simulink model "VCU_CS75_12_30_test"  (R2014a)
settings: Solver=FixedStepDiscrete  StartTime=0.0  StopTime=25  FixedStep=0.0005  RelTol=1e-3
InitFcn:
  | PID_canshu
values from neighbouring files (symbols this model uses):
  D1 = ecucoder_cal(D1)    [PID_canshu.m]
  D2 = ecucoder_cal(D2)    [PID_canshu.m]
  D3 = ecucoder_cal(D3)    [PID_canshu.m]
  ErrorLimit = ecucoder_cal(ErrorLimit)    [PID_canshu.m]
  ErrorSumMax1 = ecucoder_cal(ErrorSumMax1)    [PID_canshu.m]
  ErrorSumMax2 = ecucoder_cal(ErrorSumMax2)    [PID_canshu.m]
  ErrorSumMax3 = ecucoder_cal(ErrorSumMax3)    [PID_canshu.m]
  I1 = ecucoder_cal(I1)    [PID_canshu.m]
  I2 = ecucoder_cal(I2)    [PID_canshu.m]
  I3 = ecucoder_cal(I3)    [PID_canshu.m]
  Limit1 = ecucoder_cal(Limit1)    [PID_canshu.m]
  Limit2 = ecucoder_cal(Limit2)    [PID_canshu.m]
  P1 = ecucoder_cal(P1)    [PID_canshu.m]
  P2 = ecucoder_cal(P2)    [PID_canshu.m]
  P3 = ecucoder_cal(P3)    [PID_canshu.m]
  T_buchang = ecucoder_cal(T_buchang)    [PID_canshu.m]
undefined symbols (not defined in the file or in its folder): ecucoder_acal, I_SW01_L, LaterlAngleCommand, LDW, RemoteAcclPosition
libraries: simulink x940, ec5744lib x41
(part 9 of 31)

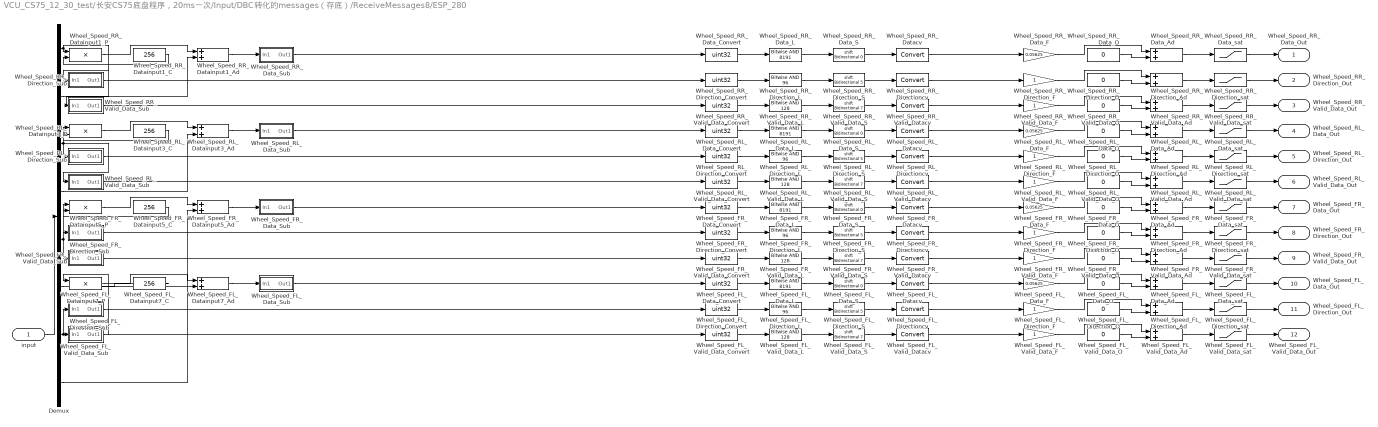
== system VCU_CS75_12_30_test/长安CS75底盘程序，20ms一次/Input/DBC转化的messages（存底）/ReceiveMessages8/ESP_280 ==
  input : Inport
  Demux : Demux  Outputs=8
  Wheel_Speed_FL_Data_Ad : Sum
  Wheel_Speed_FL_Data_Convert : DataTypeConversion  OutDataTypeStr=uint32
  Wheel_Speed_FL_Data_F : Gain  Gain=0.05625
  Wheel_Speed_FL_Data_L : simulink/Logic and Bit Operations/Bitwise Operator  logicop=AND  UseBitMask=on  BitMask=8191  BitMaskRealWorld=Stored Integer
  Wheel_Speed_FL_Data_O : Constant  Value=0  OutDataTypeStr=single
  Wheel_Speed_FL_Data_S : ArithShift
  Wheel_Speed_FL_Data_Sub : Subsystem
  Wheel_Speed_FL_Data_sat : Saturate  UpperLimit=360  LowerLimit=0
  Wheel_Speed_FL_Datacv : DataTypeConversion
  Wheel_Speed_FL_Datainput7_Ad : Sum
  Wheel_Speed_FL_Datainput7_C : Constant  Value=256
  Wheel_Speed_FL_Datainput7_P : Product
  Wheel_Speed_FL_Direction_Ad : Sum
  Wheel_Speed_FL_Direction_Convert : DataTypeConversion  OutDataTypeStr=uint32
  Wheel_Speed_FL_Direction_F : Gain
  Wheel_Speed_FL_Direction_L : simulink/Logic and Bit Operations/Bitwise Operator  logicop=AND  UseBitMask=on  BitMask=96  BitMaskRealWorld=Stored Integer
  Wheel_Speed_FL_Direction_O : Constant  Value=0  OutDataTypeStr=single
  Wheel_Speed_FL_Direction_S : ArithShift  BitShiftNumber=5
  Wheel_Speed_FL_Direction_Sub : Subsystem
  Wheel_Speed_FL_Direction_sat : Saturate  UpperLimit=3  LowerLimit=0
  Wheel_Speed_FL_Directioncv : DataTypeConversion
  Wheel_Speed_FL_Valid_Data_Ad : Sum
  Wheel_Speed_FL_Valid_Data_Convert : DataTypeConversion  OutDataTypeStr=uint32
  Wheel_Speed_FL_Valid_Data_F : Gain
  Wheel_Speed_FL_Valid_Data_L : simulink/Logic and Bit Operations/Bitwise Operator  logicop=AND  UseBitMask=on  BitMask=128  BitMaskRealWorld=Stored Integer
  Wheel_Speed_FL_Valid_Data_O : Constant  Value=0  OutDataTypeStr=single
  Wheel_Speed_FL_Valid_Data_S : ArithShift  BitShiftNumber=7
  Wheel_Speed_FL_Valid_Data_Sub : Subsystem
  Wheel_Speed_FL_Valid_Data_sat : Saturate  UpperLimit=1  LowerLimit=0
  Wheel_Speed_FL_Valid_Datacv : DataTypeConversion
  Wheel_Speed_FR_Data_Ad : Sum
  Wheel_Speed_FR_Data_Convert : DataTypeConversion  OutDataTypeStr=uint32
  Wheel_Speed_FR_Data_F : Gain  Gain=0.05625
  Wheel_Speed_FR_Data_L : simulink/Logic and Bit Operations/Bitwise Operator  logicop=AND  UseBitMask=on  BitMask=8191  BitMaskRealWorld=Stored Integer
  Wheel_Speed_FR_Data_O : Constant  Value=0  OutDataTypeStr=single
  Wheel_Speed_FR_Data_S : ArithShift
  Wheel_Speed_FR_Data_Sub : Subsystem
  Wheel_Speed_FR_Data_sat : Saturate  UpperLimit=360  LowerLimit=0
  Wheel_Speed_FR_Datacv : DataTypeConversion
  Wheel_Speed_FR_Datainput5_Ad : Sum
  Wheel_Speed_FR_Datainput5_C : Constant  Value=256
  Wheel_Speed_FR_Datainput5_P : Product
  Wheel_Speed_FR_Direction_Ad : Sum
  Wheel_Speed_FR_Direction_Convert : DataTypeConversion  OutDataTypeStr=uint32
  Wheel_Speed_FR_Direction_F : Gain
  Wheel_Speed_FR_Direction_L : simulink/Logic and Bit Operations/Bitwise Operator  logicop=AND  UseBitMask=on  BitMask=96  BitMaskRealWorld=Stored Integer
  Wheel_Speed_FR_Direction_O : Constant  Value=0  OutDataTypeStr=single
  Wheel_Speed_FR_Direction_S : ArithShift  BitShiftNumber=5
  Wheel_Speed_FR_Direction_Sub : Subsystem
  Wheel_Speed_FR_Direction_sat : Saturate  UpperLimit=3  LowerLimit=0
  Wheel_Speed_FR_Directioncv : DataTypeConversion
  Wheel_Speed_FR_Valid_Data_Ad : Sum
  Wheel_Speed_FR_Valid_Data_Convert : DataTypeConversion  OutDataTypeStr=uint32
  Wheel_Speed_FR_Valid_Data_F : Gain
  Wheel_Speed_FR_Valid_Data_L : simulink/Logic and Bit Operations/Bitwise Operator  logicop=AND  UseBitMask=on  BitMask=128  BitMaskRealWorld=Stored Integer
  Wheel_Speed_FR_Valid_Data_O : Constant  Value=0  OutDataTypeStr=single
  Wheel_Speed_FR_Valid_Data_S : ArithShift  BitShiftNumber=7
  Wheel_Speed_FR_Valid_Data_Sub : Subsystem
  Wheel_Speed_FR_Valid_Data_sat : Saturate  UpperLimit=1  LowerLimit=0
  Wheel_Speed_FR_Valid_Datacv : DataTypeConversion
  Wheel_Speed_RL_Data_Ad : Sum
  Wheel_Speed_RL_Data_Convert : DataTypeConversion  OutDataTypeStr=uint32
  Wheel_Speed_RL_Data_F : Gain  Gain=0.05625
  Wheel_Speed_RL_Data_L : simulink/Logic and Bit Operations/Bitwise Operator  logicop=AND  UseBitMask=on  BitMask=8191  BitMaskRealWorld=Stored Integer
  Wheel_Speed_RL_Data_O : Constant  Value=0  OutDataTypeStr=single
  Wheel_Speed_RL_Data_S : ArithShift
  Wheel_Speed_RL_Data_Sub : Subsystem
  Wheel_Speed_RL_Data_sat : Saturate  UpperLimit=360  LowerLimit=0
  Wheel_Speed_RL_Datacv : DataTypeConversion
  Wheel_Speed_RL_Datainput3_Ad : Sum
  Wheel_Speed_RL_Datainput3_C : Constant  Value=256
  Wheel_Speed_RL_Datainput3_P : Product
  Wheel_Speed_RL_Direction_Ad : Sum
  Wheel_Speed_RL_Direction_Convert : DataTypeConversion  OutDataTypeStr=uint32
  Wheel_Speed_RL_Direction_F : Gain
  Wheel_Speed_RL_Direction_L : simulink/Logic and Bit Operations/Bitwise Operator  logicop=AND  UseBitMask=on  BitMask=96  BitMaskRealWorld=Stored Integer
  Wheel_Speed_RL_Direction_O : Constant  Value=0  OutDataTypeStr=single
  Wheel_Speed_RL_Direction_S : ArithShift  BitShiftNumber=5
  Wheel_Speed_RL_Direction_Sub : Subsystem
  Wheel_Speed_RL_Direction_sat : Saturate  UpperLimit=3  LowerLimit=0
  Wheel_Speed_RL_Directioncv : DataTypeConversion
  Wheel_Speed_RL_Valid_Data_Ad : Sum
  Wheel_Speed_RL_Valid_Data_Convert : DataTypeConversion  OutDataTypeStr=uint32
  Wheel_Speed_RL_Valid_Data_F : Gain
  Wheel_Speed_RL_Valid_Data_L : simulink/Logic and Bit Operations/Bitwise Operator  logicop=AND  UseBitMask=on  BitMask=128  BitMaskRealWorld=Stored Integer
  Wheel_Speed_RL_Valid_Data_O : Constant  Value=0  OutDataTypeStr=single
  Wheel_Speed_RL_Valid_Data_S : ArithShift  BitShiftNumber=7
  Wheel_Speed_RL_Valid_Data_Sub : Subsystem
  Wheel_Speed_RL_Valid_Data_sat : Saturate  UpperLimit=1  LowerLimit=0
  Wheel_Speed_RL_Valid_Datacv : DataTypeConversion
  Wheel_Speed_RR_Data_Ad : Sum
  Wheel_Speed_RR_Data_Convert : DataTypeConversion  OutDataTypeStr=uint32
  Wheel_Speed_RR_Data_F : Gain  Gain=0.05625
  Wheel_Speed_RR_Data_L : simulink/Logic and Bit Operations/Bitwise Operator  logicop=AND  UseBitMask=on  BitMask=8191  BitMaskRealWorld=Stored Integer
  Wheel_Speed_RR_Data_O : Constant  Value=0  OutDataTypeStr=single
  Wheel_Speed_RR_Data_S : ArithShift
  Wheel_Speed_RR_Data_Sub : Subsystem
  Wheel_Speed_RR_Data_sat : Saturate  UpperLimit=360  LowerLimit=0
  Wheel_Speed_RR_Datacv : DataTypeConversion
  Wheel_Speed_RR_Datainput1_Ad : Sum
  Wheel_Speed_RR_Datainput1_C : Constant  Value=256
  Wheel_Speed_RR_Datainput1_P : Product
  Wheel_Speed_RR_Direction_Ad : Sum
  Wheel_Speed_RR_Direction_Convert : DataTypeConversion  OutDataTypeStr=uint32
  Wheel_Speed_RR_Direction_F : Gain
  Wheel_Speed_RR_Direction_L : simulink/Logic and Bit Operations/Bitwise Operator  logicop=AND  UseBitMask=on  BitMask=96  BitMaskRealWorld=Stored Integer
  Wheel_Speed_RR_Direction_O : Constant  Value=0  OutDataTypeStr=single
  Wheel_Speed_RR_Direction_S : ArithShift  BitShiftNumber=5
  Wheel_Speed_RR_Direction_Sub : Subsystem
  Wheel_Speed_RR_Direction_sat : Saturate  UpperLimit=3  LowerLimit=0
  Wheel_Speed_RR_Directioncv : DataTypeConversion
  Wheel_Speed_RR_Valid_Data_Ad : Sum
  Wheel_Speed_RR_Valid_Data_Convert : DataTypeConversion  OutDataTypeStr=uint32
  Wheel_Speed_RR_Valid_Data_F : Gain
  Wheel_Speed_RR_Valid_Data_L : simulink/Logic and Bit Operations/Bitwise Operator  logicop=AND  UseBitMask=on  BitMask=128  BitMaskRealWorld=Stored Integer
  Wheel_Speed_RR_Valid_Data_O : Constant  Value=0  OutDataTypeStr=single
  Wheel_Speed_RR_Valid_Data_S : ArithShift  BitShiftNumber=7
  Wheel_Speed_RR_Valid_Data_Sub : Subsystem
  Wheel_Speed_RR_Valid_Data_sat : Saturate  UpperLimit=1  LowerLimit=0
  Wheel_Speed_RR_Valid_Datacv : DataTypeConversion
  Wheel_Speed_RR_Data_Out : Outport
  Wheel_Speed_RR_Direction_Out : Outport  Port=2
  Wheel_Speed_RR_Valid_Data_Out : Outport  Port=3
  Wheel_Speed_RL_Data_Out : Outport  Port=4
  Wheel_Speed_RL_Direction_Out : Outport  Port=5
  Wheel_Speed_RL_Valid_Data_Out : Outport  Port=6
  Wheel_Speed_FR_Data_Out : Outport  Port=7
  Wheel_Speed_FR_Direction_Out : Outport  Port=8
  Wheel_Speed_FR_Valid_Data_Out : Outport  Port=9
  Wheel_Speed_FL_Data_Out : Outport  Port=10
  Wheel_Speed_FL_Direction_Out : Outport  Port=11
  Wheel_Speed_FL_Valid_Data_Out : Outport  Port=12
  wires:
  input/1 -> Demux/1
  Wheel_Speed_FL_Valid_Datacv/1 -> Wheel_Speed_FL_Valid_Data_F/1
  Wheel_Speed_FL_Valid_Data_S/1 -> Wheel_Speed_FL_Valid_Datacv/1
  Wheel_Speed_FL_Valid_Data_L/1 -> Wheel_Speed_FL_Valid_Data_S/1
  Wheel_Speed_FL_Valid_Data_Convert/1 -> Wheel_Speed_FL_Valid_Data_L/1
  Wheel_Speed_FL_Valid_Data_Sub/1(Out1) -> Wheel_Speed_FL_Valid_Data_Convert/1
  Wheel_Speed_FL_Valid_Data_sat/1 -> Wheel_Speed_FL_Valid_Data_Out/1
  Wheel_Speed_FL_Valid_Data_Ad/1 -> Wheel_Speed_FL_Valid_Data_sat/1
  Wheel_Speed_FL_Valid_Data_O/1 -> Wheel_Speed_FL_Valid_Data_Ad/2
  Wheel_Speed_FL_Valid_Data_F/1 -> Wheel_Speed_FL_Valid_Data_Ad/1
  Wheel_Speed_FL_Directioncv/1 -> Wheel_Speed_FL_Direction_F/1
  Wheel_Speed_FL_Direction_S/1 -> Wheel_Speed_FL_Directioncv/1
  Wheel_Speed_FL_Direction_L/1 -> Wheel_Speed_FL_Direction_S/1
  Wheel_Speed_FL_Direction_Convert/1 -> Wheel_Speed_FL_Direction_L/1
  Wheel_Speed_FL_Direction_Sub/1(Out1) -> Wheel_Speed_FL_Direction_Convert/1
  Wheel_Speed_FL_Direction_sat/1 -> Wheel_Speed_FL_Direction_Out/1
  Wheel_Speed_FL_Direction_Ad/1 -> Wheel_Speed_FL_Direction_sat/1
  Wheel_Speed_FL_Direction_O/1 -> Wheel_Speed_FL_Direction_Ad/2
  Wheel_Speed_FL_Direction_F/1 -> Wheel_Speed_FL_Direction_Ad/1
  Wheel_Speed_FL_Datacv/1 -> Wheel_Speed_FL_Data_F/1
  Wheel_Speed_FL_Data_S/1 -> Wheel_Speed_FL_Datacv/1
  Wheel_Speed_FL_Data_L/1 -> Wheel_Speed_FL_Data_S/1
  Wheel_Speed_FL_Data_Convert/1 -> Wheel_Speed_FL_Data_L/1
  Wheel_Speed_FL_Data_Sub/1(Out1) -> Wheel_Speed_FL_Data_Convert/1
  Wheel_Speed_FL_Datainput7_Ad/1 -> Wheel_Speed_FL_Data_Sub/1(In1)
  Demux/8 -> Wheel_Speed_FL_Datainput7_Ad/2
  Wheel_Speed_FL_Datainput7_P/1 -> Wheel_Speed_FL_Datainput7_Ad/1
  Wheel_Speed_FL_Datainput7_C/1 -> Wheel_Speed_FL_Datainput7_P/2
  Demux/7 -> Wheel_Speed_FL_Valid_Data_Sub/1(In1), Wheel_Speed_FL_Direction_Sub/1(In1), Wheel_Speed_FL_Datainput7_P/1
  Wheel_Speed_FL_Data_sat/1 -> Wheel_Speed_FL_Data_Out/1
  Wheel_Speed_FL_Data_Ad/1 -> Wheel_Speed_FL_Data_sat/1
  Wheel_Speed_FL_Data_O/1 -> Wheel_Speed_FL_Data_Ad/2
  Wheel_Speed_FL_Data_F/1 -> Wheel_Speed_FL_Data_Ad/1
  Wheel_Speed_FR_Valid_Datacv/1 -> Wheel_Speed_FR_Valid_Data_F/1
  Wheel_Speed_FR_Valid_Data_S/1 -> Wheel_Speed_FR_Valid_Datacv/1
  Wheel_Speed_FR_Valid_Data_L/1 -> Wheel_Speed_FR_Valid_Data_S/1
  Wheel_Speed_FR_Valid_Data_Convert/1 -> Wheel_Speed_FR_Valid_Data_L/1
  Wheel_Speed_FR_Valid_Data_Sub/1(Out1) -> Wheel_Speed_FR_Valid_Data_Convert/1
  Wheel_Speed_FR_Valid_Data_sat/1 -> Wheel_Speed_FR_Valid_Data_Out/1
  Wheel_Speed_FR_Valid_Data_Ad/1 -> Wheel_Speed_FR_Valid_Data_sat/1
  Wheel_Speed_FR_Valid_Data_O/1 -> Wheel_Speed_FR_Valid_Data_Ad/2
  Wheel_Speed_FR_Valid_Data_F/1 -> Wheel_Speed_FR_Valid_Data_Ad/1
  Wheel_Speed_FR_Directioncv/1 -> Wheel_Speed_FR_Direction_F/1
  Wheel_Speed_FR_Direction_S/1 -> Wheel_Speed_FR_Directioncv/1
  Wheel_Speed_FR_Direction_L/1 -> Wheel_Speed_FR_Direction_S/1
  Wheel_Speed_FR_Direction_Convert/1 -> Wheel_Speed_FR_Direction_L/1
  Wheel_Speed_FR_Direction_Sub/1(Out1) -> Wheel_Speed_FR_Direction_Convert/1
  Wheel_Speed_FR_Direction_sat/1 -> Wheel_Speed_FR_Direction_Out/1
  Wheel_Speed_FR_Direction_Ad/1 -> Wheel_Speed_FR_Direction_sat/1
  Wheel_Speed_FR_Direction_O/1 -> Wheel_Speed_FR_Direction_Ad/2
  Wheel_Speed_FR_Direction_F/1 -> Wheel_Speed_FR_Direction_Ad/1
  Wheel_Speed_FR_Datacv/1 -> Wheel_Speed_FR_Data_F/1
  Wheel_Speed_FR_Data_S/1 -> Wheel_Speed_FR_Datacv/1
  Wheel_Speed_FR_Data_L/1 -> Wheel_Speed_FR_Data_S/1
  Wheel_Speed_FR_Data_Convert/1 -> Wheel_Speed_FR_Data_L/1
  Wheel_Speed_FR_Data_Sub/1(Out1) -> Wheel_Speed_FR_Data_Convert/1
  Wheel_Speed_FR_Datainput5_Ad/1 -> Wheel_Speed_FR_Data_Sub/1(In1)
  Demux/6 -> Wheel_Speed_FR_Datainput5_Ad/2
  Wheel_Speed_FR_Datainput5_P/1 -> Wheel_Speed_FR_Datainput5_Ad/1
  Wheel_Speed_FR_Datainput5_C/1 -> Wheel_Speed_FR_Datainput5_P/2
  Demux/5 -> Wheel_Speed_FR_Valid_Data_Sub/1(In1), Wheel_Speed_FR_Direction_Sub/1(In1), Wheel_Speed_FR_Datainput5_P/1
  Wheel_Speed_FR_Data_sat/1 -> Wheel_Speed_FR_Data_Out/1
  Wheel_Speed_FR_Data_Ad/1 -> Wheel_Speed_FR_Data_sat/1
  Wheel_Speed_FR_Data_O/1 -> Wheel_Speed_FR_Data_Ad/2
  Wheel_Speed_FR_Data_F/1 -> Wheel_Speed_FR_Data_Ad/1
  Wheel_Speed_RL_Valid_Datacv/1 -> Wheel_Speed_RL_Valid_Data_F/1
  Wheel_Speed_RL_Valid_Data_S/1 -> Wheel_Speed_RL_Valid_Datacv/1
  Wheel_Speed_RL_Valid_Data_L/1 -> Wheel_Speed_RL_Valid_Data_S/1
  Wheel_Speed_RL_Valid_Data_Convert/1 -> Wheel_Speed_RL_Valid_Data_L/1
  Wheel_Speed_RL_Valid_Data_Sub/1(Out1) -> Wheel_Speed_RL_Valid_Data_Convert/1
  Wheel_Speed_RL_Valid_Data_sat/1 -> Wheel_Speed_RL_Valid_Data_Out/1
  Wheel_Speed_RL_Valid_Data_Ad/1 -> Wheel_Speed_RL_Valid_Data_sat/1
  Wheel_Speed_RL_Valid_Data_O/1 -> Wheel_Speed_RL_Valid_Data_Ad/2
  Wheel_Speed_RL_Valid_Data_F/1 -> Wheel_Speed_RL_Valid_Data_Ad/1
  Wheel_Speed_RL_Directioncv/1 -> Wheel_Speed_RL_Direction_F/1
  Wheel_Speed_RL_Direction_S/1 -> Wheel_Speed_RL_Directioncv/1
  Wheel_Speed_RL_Direction_L/1 -> Wheel_Speed_RL_Direction_S/1
  Wheel_Speed_RL_Direction_Convert/1 -> Wheel_Speed_RL_Direction_L/1
  Wheel_Speed_RL_Direction_Sub/1(Out1) -> Wheel_Speed_RL_Direction_Convert/1
  Wheel_Speed_RL_Direction_sat/1 -> Wheel_Speed_RL_Direction_Out/1
  Wheel_Speed_RL_Direction_Ad/1 -> Wheel_Speed_RL_Direction_sat/1
  Wheel_Speed_RL_Direction_O/1 -> Wheel_Speed_RL_Direction_Ad/2
  Wheel_Speed_RL_Direction_F/1 -> Wheel_Speed_RL_Direction_Ad/1
  Wheel_Speed_RL_Datacv/1 -> Wheel_Speed_RL_Data_F/1
  Wheel_Speed_RL_Data_S/1 -> Wheel_Speed_RL_Datacv/1
  Wheel_Speed_RL_Data_L/1 -> Wheel_Speed_RL_Data_S/1
  Wheel_Speed_RL_Data_Convert/1 -> Wheel_Speed_RL_Data_L/1
  Wheel_Speed_RL_Data_Sub/1(Out1) -> Wheel_Speed_RL_Data_Convert/1
  Wheel_Speed_RL_Datainput3_Ad/1 -> Wheel_Speed_RL_Data_Sub/1(In1)
  Demux/4 -> Wheel_Speed_RL_Datainput3_Ad/2
  Wheel_Speed_RL_Datainput3_P/1 -> Wheel_Speed_RL_Datainput3_Ad/1
  Wheel_Speed_RL_Datainput3_C/1 -> Wheel_Speed_RL_Datainput3_P/2
  Demux/3 -> Wheel_Speed_RL_Valid_Data_Sub/1(In1), Wheel_Speed_RL_Direction_Sub/1(In1), Wheel_Speed_RL_Datainput3_P/1
  Wheel_Speed_RL_Data_sat/1 -> Wheel_Speed_RL_Data_Out/1
  Wheel_Speed_RL_Data_Ad/1 -> Wheel_Speed_RL_Data_sat/1
  Wheel_Speed_RL_Data_O/1 -> Wheel_Speed_RL_Data_Ad/2
  Wheel_Speed_RL_Data_F/1 -> Wheel_Speed_RL_Data_Ad/1
  Wheel_Speed_RR_Valid_Datacv/1 -> Wheel_Speed_RR_Valid_Data_F/1
  Wheel_Speed_RR_Valid_Data_S/1 -> Wheel_Speed_RR_Valid_Datacv/1
  Wheel_Speed_RR_Valid_Data_L/1 -> Wheel_Speed_RR_Valid_Data_S/1
  Wheel_Speed_RR_Valid_Data_Convert/1 -> Wheel_Speed_RR_Valid_Data_L/1
  Wheel_Speed_RR_Valid_Data_Sub/1(Out1) -> Wheel_Speed_RR_Valid_Data_Convert/1
  Wheel_Speed_RR_Valid_Data_sat/1 -> Wheel_Speed_RR_Valid_Data_Out/1
  Wheel_Speed_RR_Valid_Data_Ad/1 -> Wheel_Speed_RR_Valid_Data_sat/1
  Wheel_Speed_RR_Valid_Data_O/1 -> Wheel_Speed_RR_Valid_Data_Ad/2
  Wheel_Speed_RR_Valid_Data_F/1 -> Wheel_Speed_RR_Valid_Data_Ad/1
  Wheel_Speed_RR_Directioncv/1 -> Wheel_Speed_RR_Direction_F/1
  Wheel_Speed_RR_Direction_S/1 -> Wheel_Speed_RR_Directioncv/1
  Wheel_Speed_RR_Direction_L/1 -> Wheel_Speed_RR_Direction_S/1
  Wheel_Speed_RR_Direction_Convert/1 -> Wheel_Speed_RR_Direction_L/1
  Wheel_Speed_RR_Direction_Sub/1(Out1) -> Wheel_Speed_RR_Direction_Convert/1
  Wheel_Speed_RR_Direction_sat/1 -> Wheel_Speed_RR_Direction_Out/1
  Wheel_Speed_RR_Direction_Ad/1 -> Wheel_Speed_RR_Direction_sat/1
  Wheel_Speed_RR_Direction_O/1 -> Wheel_Speed_RR_Direction_Ad/2
  Wheel_Speed_RR_Direction_F/1 -> Wheel_Speed_RR_Direction_Ad/1
  Wheel_Speed_RR_Datacv/1 -> Wheel_Speed_RR_Data_F/1
  Wheel_Speed_RR_Data_S/1 -> Wheel_Speed_RR_Datacv/1
  Wheel_Speed_RR_Data_L/1 -> Wheel_Speed_RR_Data_S/1
  Wheel_Speed_RR_Data_Convert/1 -> Wheel_Speed_RR_Data_L/1
  Wheel_Speed_RR_Data_Sub/1(Out1) -> Wheel_Speed_RR_Data_Convert/1
  Wheel_Speed_RR_Datainput1_Ad/1 -> Wheel_Speed_RR_Data_Sub/1(In1)
  Demux/2 -> Wheel_Speed_RR_Datainput1_Ad/2
  Wheel_Speed_RR_Datainput1_P/1 -> Wheel_Speed_RR_Datainput1_Ad/1
  Wheel_Speed_RR_Datainput1_C/1 -> Wheel_Speed_RR_Datainput1_P/2
  Demux/1 -> Wheel_Speed_RR_Valid_Data_Sub/1(In1), Wheel_Speed_RR_Direction_Sub/1(In1), Wheel_Speed_RR_Datainput1_P/1
  Wheel_Speed_RR_Data_sat/1 -> Wheel_Speed_RR_Data_Out/1
  Wheel_Speed_RR_Data_Ad/1 -> Wheel_Speed_RR_Data_sat/1
  Wheel_Speed_RR_Data_O/1 -> Wheel_Speed_RR_Data_Ad/2
  Wheel_Speed_RR_Data_F/1 -> Wheel_Speed_RR_Data_Ad/1

== system VCU_CS75_12_30_test/长安CS75底盘程序，20ms一次/Input/DBC转化的messages（存底）/ReceiveMessages9/ESP_281 ==
  input : Inport
  Demux : Demux  Outputs=8
  ESP_ABSActiveStatus_Ad : Sum
  ESP_ABSActiveStatus_Convert : DataTypeConversion  OutDataTypeStr=uint32
  ESP_ABSActiveStatus_F : Gain
  ESP_ABSActiveStatus_L : simulink/Logic and Bit Operations/Bitwise Operator  logicop=AND  UseBitMask=on  BitMask=128  BitMaskRealWorld=Stored Integer
  ESP_ABSActiveStatus_O : Constant  Value=0  OutDataTypeStr=single
  ESP_ABSActiveStatus_S : ArithShift  BitShiftNumber=7
  ESP_ABSActiveStatus_Sub : Subsystem
  ESP_ABSActiveStatus_sat : Saturate  UpperLimit=1  LowerLimit=0
  ESP_ABSActiveStatuscv : DataTypeConversion
  ESP_ABSFailStatus_Ad : Sum
  ESP_ABSFailStatus_Convert : DataTypeConversion  OutDataTypeStr=uint32
  ESP_ABSFailStatus_F : Gain
  ESP_ABSFailStatus_L : simulink/Logic and Bit Operations/Bitwise Operator  logicop=AND  UseBitMask=on  BitMask=8  BitMaskRealWorld=Stored Integer
  ESP_ABSFailStatus_O : Constant  Value=0  OutDataTypeStr=single
  ESP_ABSFailStatus_S : ArithShift  BitShiftNumber=3
  ESP_ABSFailStatus_Sub : Subsystem
  ESP_ABSFailStatus_sat : Saturate  UpperLimit=1  LowerLimit=0
  ESP_ABSFailStatuscv : DataTypeConversion
  ESP_BrakePedalStatus_Ad : Sum
  ESP_BrakePedalStatus_Convert : DataTypeConversion  OutDataTypeStr=uint32
  ESP_BrakePedalStatus_F : Gain
  ESP_BrakePedalStatus_L : simulink/Logic and Bit Operations/Bitwise Operator  logicop=AND  UseBitMask=on  BitMask=96  BitMaskRealWorld=Stored Integer
  ESP_BrakePedalStatus_O : Constant  Value=0  OutDataTypeStr=single
  ESP_BrakePedalStatus_S : ArithShift  BitShiftNumber=5
  ESP_BrakePedalStatus_Sub : Subsystem
  ESP_BrakePedalStatus_sat : Saturate  UpperLimit=3  LowerLimit=0
  ESP_BrakePedalStatuscv : DataTypeConversion
  ESP_Checksum_Ad : Sum
  ESP_Checksum_Convert : DataTypeConversion  OutDataTypeStr=uint32
  ESP_Checksum_F : Gain
  ESP_Checksum_L : simulink/Logic and Bit Operations/Bitwise Operator  logicop=AND  UseBitMask=on  BitMask=255  BitMaskRealWorld=Stored Integer
  ESP_Checksum_O : Constant  Value=0  OutDataTypeStr=single
  ESP_Checksum_S : ArithShift
  ESP_Checksum_Sub : Subsystem
  ESP_Checksum_sat : Saturate  UpperLimit=255  LowerLimit=0
  ESP_Checksumcv : DataTypeConversion
  ESP_EBDFailStatus_Ad : Sum
  ESP_EBDFailStatus_Convert : DataTypeConversion  OutDataTypeStr=uint32
  ESP_EBDFailStatus_F : Gain
  ESP_EBDFailStatus_L : simulink/Logic and Bit Operations/Bitwise Operator  logicop=AND  UseBitMask=on  BitMask=4  BitMaskRealWorld=Stored Integer
  ESP_EBDFailStatus_O : Constant  Value=0  OutDataTypeStr=single
  ESP_EBDFailStatus_S : ArithShift  BitShiftNumber=2
  ESP_EBDFailStatus_Sub : Subsystem
  ESP_EBDFailStatus_sat : Saturate  UpperLimit=1  LowerLimit=0
  ESP_EBDFailStatuscv : DataTypeConversion
  ESP_ESPActiveStatus_Ad : Sum
  ESP_ESPActiveStatus_Convert : DataTypeConversion  OutDataTypeStr=uint32
  ESP_ESPActiveStatus_F : Gain
  ESP_ESPActiveStatus_L : simulink/Logic and Bit Operations/Bitwise Operator  logicop=AND  UseBitMask=on  BitMask=1  BitMaskRealWorld=Stored Integer
  ESP_ESPActiveStatus_O : Constant  Value=0  OutDataTypeStr=single
  ESP_ESPActiveStatus_S : ArithShift
  ESP_ESPActiveStatus_Sub : Subsystem
  ESP_ESPActiveStatus_sat : Saturate  UpperLimit=1  LowerLimit=0
  ESP_ESPActiveStatuscv : DataTypeConversion
  ESP_ESPFailStatus_Ad : Sum
  ESP_ESPFailStatus_Convert : DataTypeConversion  OutDataTypeStr=uint32
  ESP_ESPFailStatus_F : Gain
  ESP_ESPFailStatus_L : simulink/Logic and Bit Operations/Bitwise Operator  logicop=AND  UseBitMask=on  BitMask=16  BitMaskRealWorld=Stored Integer
  ESP_ESPFailStatus_O : Constant  Value=0  OutDataTypeStr=single
  ESP_ESPFailStatus_S : ArithShift  BitShiftNumber=4
  ESP_ESPFailStatus_Sub : Subsystem
  ESP_ESPFailStatus_sat : Saturate  UpperLimit=1  LowerLimit=0
  ESP_ESPFailStatuscv : DataTypeConversion
  ESP_ESPSwitchStatus_Ad : Sum
  ESP_ESPSwitchStatus_Convert : DataTypeConversion  OutDataTypeStr=uint32
  ESP_ESPSwitchStatus_F : Gain
  ESP_ESPSwitchStatus_L : simulink/Logic and Bit Operations/Bitwise Operator  logicop=AND  UseBitMask=on  BitMask=2  BitMaskRealWorld=Stored Integer
  ESP_ESPSwitchStatus_O : Constant  Value=0  OutDataTypeStr=single
  ESP_ESPSwitchStatus_S : ArithShift  BitShiftNumber=1
  ESP_ESPSwitchStatus_Sub : Subsystem
  ESP_ESPSwitchStatus_sat : Saturate  UpperLimit=1  LowerLimit=0
  ESP_ESPSwitchStatuscv : DataTypeConversion
  ESP_RollingCounter_Ad : Sum
  ESP_RollingCounter_Convert : DataTypeConversion  OutDataTypeStr=uint32
  ESP_RollingCounter_F : Gain
  ESP_RollingCounter_L : simulink/Logic and Bit Operations/Bitwise Operator  logicop=AND  UseBitMask=on  BitMask=15  BitMaskRealWorld=Stored Integer
  ESP_RollingCounter_O : Constant  Value=0  OutDataTypeStr=single
  ESP_RollingCounter_S : ArithShift
  ESP_RollingCounter_Sub : Subsystem
  ESP_RollingCounter_sat : Saturate  UpperLimit=15  LowerLimit=0
  ESP_RollingCountercv : DataTypeConversion
  ESP_VehicleSpeed_Ad : Sum
  ESP_VehicleSpeed_Convert : DataTypeConversion  OutDataTypeStr=uint32
  ESP_VehicleSpeed_F : Gain  Gain=0.05625
  ESP_VehicleSpeed_L : simulink/Logic and Bit Operations/Bitwise Operator  logicop=AND  UseBitMask=on  BitMask=8191  BitMaskRealWorld=Stored Integer
  ESP_VehicleSpeed_O : Constant  Value=0  OutDataTypeStr=single
  ESP_VehicleSpeed_S : ArithShift
  ESP_VehicleSpeed_Status_Ad : Sum
  ESP_VehicleSpeed_Status_Convert : DataTypeConversion  OutDataTypeStr=uint32
  ESP_VehicleSpeed_Status_F : Gain
  ESP_VehicleSpeed_Status_L : simulink/Logic and Bit Operations/Bitwise Operator  logicop=AND  UseBitMask=on  BitMask=32  BitMaskRealWorld=Stored Integer
  ESP_VehicleSpeed_Status_O : Constant  Value=0  OutDataTypeStr=single
  ESP_VehicleSpeed_Status_S : ArithShift  BitShiftNumber=5
  ESP_VehicleSpeed_Status_Sub : Subsystem
  ESP_VehicleSpeed_Status_sat : Saturate  UpperLimit=1  LowerLimit=0
  ESP_VehicleSpeed_Statuscv : DataTypeConversion
  ESP_VehicleSpeed_Sub : Subsystem
  ESP_VehicleSpeed_sat : Saturate  UpperLimit=360  LowerLimit=0
  ESP_VehicleSpeedcv : DataTypeConversion
  ESP_VehicleSpeedinput5_Ad : Sum
  ESP_VehicleSpeedinput5_C : Constant  Value=256
  ESP_VehicleSpeedinput5_P : Product
  ESP_ESPActiveStatus_Out : Outport
  ESP_ESPSwitchStatus_Out : Outport  Port=2
  ESP_EBDFailStatus_Out : Outport  Port=3
  ESP_ABSFailStatus_Out : Outport  Port=4
  ESP_ESPFailStatus_Out : Outport  Port=5
  ESP_ABSActiveStatus_Out : Outport  Port=6
  ESP_VehicleSpeed_Out : Outport  Port=7
  ESP_VehicleSpeed_Status_Out : Outport  Port=8
  ESP_RollingCounter_Out : Outport  Port=9
  ESP_BrakePedalStatus_Out : Outport  Port=10
  ESP_Checksum_Out : Outport  Port=11
  wires:
  input/1 -> Demux/1
  ESP_Checksumcv/1 -> ESP_Checksum_F/1
  ESP_Checksum_S/1 -> ESP_Checksumcv/1
  ESP_Checksum_L/1 -> ESP_Checksum_S/1
  ESP_Checksum_Convert/1 -> ESP_Checksum_L/1
  ESP_Checksum_Sub/1(Out1) -> ESP_Checksum_Convert/1
  Demux/8 -> ESP_Checksum_Sub/1(In1)
  ESP_Checksum_sat/1 -> ESP_Checksum_Out/1
  ESP_Checksum_Ad/1 -> ESP_Checksum_sat/1
  ESP_Checksum_O/1 -> ESP_Checksum_Ad/2
  ESP_Checksum_F/1 -> ESP_Checksum_Ad/1
  ESP_BrakePedalStatuscv/1 -> ESP_BrakePedalStatus_F/1
  ESP_BrakePedalStatus_S/1 -> ESP_BrakePedalStatuscv/1
  ESP_BrakePedalStatus_L/1 -> ESP_BrakePedalStatus_S/1
  ESP_BrakePedalStatus_Convert/1 -> ESP_BrakePedalStatus_L/1
  ESP_BrakePedalStatus_Sub/1(Out1) -> ESP_BrakePedalStatus_Convert/1
  ESP_BrakePedalStatus_sat/1 -> ESP_BrakePedalStatus_Out/1
  ESP_BrakePedalStatus_Ad/1 -> ESP_BrakePedalStatus_sat/1
  ESP_BrakePedalStatus_O/1 -> ESP_BrakePedalStatus_Ad/2
  ESP_BrakePedalStatus_F/1 -> ESP_BrakePedalStatus_Ad/1
  ESP_RollingCountercv/1 -> ESP_RollingCounter_F/1
  ESP_RollingCounter_S/1 -> ESP_RollingCountercv/1
  ESP_RollingCounter_L/1 -> ESP_RollingCounter_S/1
  ESP_RollingCounter_Convert/1 -> ESP_RollingCounter_L/1
  ESP_RollingCounter_Sub/1(Out1) -> ESP_RollingCounter_Convert/1
  Demux/7 -> ESP_BrakePedalStatus_Sub/1(In1), ESP_RollingCounter_Sub/1(In1)
  ESP_RollingCounter_sat/1 -> ESP_RollingCounter_Out/1
  ESP_RollingCounter_Ad/1 -> ESP_RollingCounter_sat/1
  ESP_RollingCounter_O/1 -> ESP_RollingCounter_Ad/2
  ESP_RollingCounter_F/1 -> ESP_RollingCounter_Ad/1
  ESP_VehicleSpeed_Statuscv/1 -> ESP_VehicleSpeed_Status_F/1
  ESP_VehicleSpeed_Status_S/1 -> ESP_VehicleSpeed_Statuscv/1
  ESP_VehicleSpeed_Status_L/1 -> ESP_VehicleSpeed_Status_S/1
  ESP_VehicleSpeed_Status_Convert/1 -> ESP_VehicleSpeed_Status_L/1
  ESP_VehicleSpeed_Status_Sub/1(Out1) -> ESP_VehicleSpeed_Status_Convert/1
  ESP_VehicleSpeed_Status_sat/1 -> ESP_VehicleSpeed_Status_Out/1
  ESP_VehicleSpeed_Status_Ad/1 -> ESP_VehicleSpeed_Status_sat/1
  ESP_VehicleSpeed_Status_O/1 -> ESP_VehicleSpeed_Status_Ad/2
  ESP_VehicleSpeed_Status_F/1 -> ESP_VehicleSpeed_Status_Ad/1
  ESP_VehicleSpeedcv/1 -> ESP_VehicleSpeed_F/1
  ESP_VehicleSpeed_S/1 -> ESP_VehicleSpeedcv/1
  ESP_VehicleSpeed_L/1 -> ESP_VehicleSpeed_S/1
  ESP_VehicleSpeed_Convert/1 -> ESP_VehicleSpeed_L/1
  ESP_VehicleSpeed_Sub/1(Out1) -> ESP_VehicleSpeed_Convert/1
  ESP_VehicleSpeedinput5_Ad/1 -> ESP_VehicleSpeed_Sub/1(In1)
  Demux/6 -> ESP_VehicleSpeedinput5_Ad/2
  ESP_VehicleSpeedinput5_P/1 -> ESP_VehicleSpeedinput5_Ad/1
  ESP_VehicleSpeedinput5_C/1 -> ESP_VehicleSpeedinput5_P/2
  Demux/5 -> ESP_VehicleSpeed_Status_Sub/1(In1), ESP_VehicleSpeedinput5_P/1
  ESP_VehicleSpeed_sat/1 -> ESP_VehicleSpeed_Out/1
  ESP_VehicleSpeed_Ad/1 -> ESP_VehicleSpeed_sat/1
  ESP_VehicleSpeed_O/1 -> ESP_VehicleSpeed_Ad/2
  ESP_VehicleSpeed_F/1 -> ESP_VehicleSpeed_Ad/1
  ESP_ABSActiveStatuscv/1 -> ESP_ABSActiveStatus_F/1
  ESP_ABSActiveStatus_S/1 -> ESP_ABSActiveStatuscv/1
  ESP_ABSActiveStatus_L/1 -> ESP_ABSActiveStatus_S/1
  ESP_ABSActiveStatus_Convert/1 -> ESP_ABSActiveStatus_L/1
  ESP_ABSActiveStatus_Sub/1(Out1) -> ESP_ABSActiveStatus_Convert/1
  ESP_ABSActiveStatus_sat/1 -> ESP_ABSActiveStatus_Out/1
  ESP_ABSActiveStatus_Ad/1 -> ESP_ABSActiveStatus_sat/1
  ESP_ABSActiveStatus_O/1 -> ESP_ABSActiveStatus_Ad/2
  ESP_ABSActiveStatus_F/1 -> ESP_ABSActiveStatus_Ad/1
  ESP_ESPFailStatuscv/1 -> ESP_ESPFailStatus_F/1
  ESP_ESPFailStatus_S/1 -> ESP_ESPFailStatuscv/1
  ESP_ESPFailStatus_L/1 -> ESP_ESPFailStatus_S/1
  ESP_ESPFailStatus_Convert/1 -> ESP_ESPFailStatus_L/1
  ESP_ESPFailStatus_Sub/1(Out1) -> ESP_ESPFailStatus_Convert/1
  ESP_ESPFailStatus_sat/1 -> ESP_ESPFailStatus_Out/1
  ESP_ESPFailStatus_Ad/1 -> ESP_ESPFailStatus_sat/1
  ESP_ESPFailStatus_O/1 -> ESP_ESPFailStatus_Ad/2
  ESP_ESPFailStatus_F/1 -> ESP_ESPFailStatus_Ad/1
  ESP_ABSFailStatuscv/1 -> ESP_ABSFailStatus_F/1
  ESP_ABSFailStatus_S/1 -> ESP_ABSFailStatuscv/1
  ESP_ABSFailStatus_L/1 -> ESP_ABSFailStatus_S/1
  ESP_ABSFailStatus_Convert/1 -> ESP_ABSFailStatus_L/1
  ESP_ABSFailStatus_Sub/1(Out1) -> ESP_ABSFailStatus_Convert/1
  ESP_ABSFailStatus_sat/1 -> ESP_ABSFailStatus_Out/1
  ESP_ABSFailStatus_Ad/1 -> ESP_ABSFailStatus_sat/1
  ESP_ABSFailStatus_O/1 -> ESP_ABSFailStatus_Ad/2
  ESP_ABSFailStatus_F/1 -> ESP_ABSFailStatus_Ad/1
  ESP_EBDFailStatuscv/1 -> ESP_EBDFailStatus_F/1
  ESP_EBDFailStatus_S/1 -> ESP_EBDFailStatuscv/1
  ESP_EBDFailStatus_L/1 -> ESP_EBDFailStatus_S/1
  ESP_EBDFailStatus_Convert/1 -> ESP_EBDFailStatus_L/1
  ESP_EBDFailStatus_Sub/1(Out1) -> ESP_EBDFailStatus_Convert/1
  ESP_EBDFailStatus_sat/1 -> ESP_EBDFailStatus_Out/1
  ESP_EBDFailStatus_Ad/1 -> ESP_EBDFailStatus_sat/1
  ESP_EBDFailStatus_O/1 -> ESP_EBDFailStatus_Ad/2
  ESP_EBDFailStatus_F/1 -> ESP_EBDFailStatus_Ad/1
  ESP_ESPSwitchStatuscv/1 -> ESP_ESPSwitchStatus_F/1
  ESP_ESPSwitchStatus_S/1 -> ESP_ESPSwitchStatuscv/1
  ESP_ESPSwitchStatus_L/1 -> ESP_ESPSwitchStatus_S/1
  ESP_ESPSwitchStatus_Convert/1 -> ESP_ESPSwitchStatus_L/1
  ESP_ESPSwitchStatus_Sub/1(Out1) -> ESP_ESPSwitchStatus_Convert/1
  ESP_ESPSwitchStatus_sat/1 -> ESP_ESPSwitchStatus_Out/1
  ESP_ESPSwitchStatus_Ad/1 -> ESP_ESPSwitchStatus_sat/1
  ESP_ESPSwitchStatus_O/1 -> ESP_ESPSwitchStatus_Ad/2
  ESP_ESPSwitchStatus_F/1 -> ESP_ESPSwitchStatus_Ad/1
  ESP_ESPActiveStatuscv/1 -> ESP_ESPActiveStatus_F/1
  ESP_ESPActiveStatus_S/1 -> ESP_ESPActiveStatuscv/1
  ESP_ESPActiveStatus_L/1 -> ESP_ESPActiveStatus_S/1
  ESP_ESPActiveStatus_Convert/1 -> ESP_ESPActiveStatus_L/1
  ESP_ESPActiveStatus_Sub/1(Out1) -> ESP_ESPActiveStatus_Convert/1
  Demux/1 -> ESP_ABSActiveStatus_Sub/1(In1), ESP_ESPFailStatus_Sub/1(In1), ESP_ABSFailStatus_Sub/1(In1), ESP_EBDFailStatus_Sub/1(In1), ESP_ESPSwitchStatus_Sub/1(In1), ESP_ESPActiveStatus_Sub/1(In1)
  ESP_ESPActiveStatus_sat/1 -> ESP_ESPActiveStatus_Out/1
  ESP_ESPActiveStatus_Ad/1 -> ESP_ESPActiveStatus_sat/1
  ESP_ESPActiveStatus_O/1 -> ESP_ESPActiveStatus_Ad/2
  ESP_ESPActiveStatus_F/1 -> ESP_ESPActiveStatus_Ad/1

== system VCU_CS75_12_30_test/长安CS75底盘程序，20ms一次/Output/CAN0_Tx/to502/VCU2IPC502 ==
  BrakePedalState_in : Inport
  Steering_Angle_Feedback_in : Inport  Port=2
  Steering_feedback_in : Inport  Port=3
  Wheel_Speed_RR_Feedback_in : Inport  Port=4
  Wheel_Speed_RL_Feedback_in : Inport  Port=5
  Wheel_Speed_FR_Feedback_in : Inport  Port=6
  Wheel_Speed_FL_Feedback_in : Inport  Port=7
  BrakePedalState : Subsystem
  Conv{1..8} (8 alike) : DataTypeConversion
  Steering_Angle_Feedback : Subsystem
  Steering_feedback : Subsystem
  VCU2IPC502_DLC : Constant  Value=8  OutDataTypeStr=uint8
  VCU2IPC502_DLC_Out : Terminator
  VCU2IPC502_ID : Constant  Value=1282  OutDataTypeStr=single
  VCU2IPC502_ID_Out : Terminator
  VCU2IPC502_mux : Mux  Inputs=8
  Wheel_Speed_FL_Feedback : Subsystem
  Wheel_Speed_FR_Feedback : Subsystem
  Wheel_Speed_RL_Feedback : Subsystem
  Wheel_Speed_RR_Feedback : Subsystem
  or{1..8} (8 alike) : simulink/Logic and Bit Operations/Bitwise Operator  logicop=OR  UseBitMask=off  NumInputPorts=7  BitMask=bin2dec('11011001')  BitMaskRealWorld=Stored Integer
  output : Outport
  wires:
  VCU2IPC502_mux/1 -> output/1
  BrakePedalState/1(output1) -> or1/1
  BrakePedalState/2(output2) -> or2/1
  BrakePedalState/3(output3) -> or3/1
  BrakePedalState/4(output4) -> or4/1
  BrakePedalState/5(output5) -> or5/1
  BrakePedalState/6(output6) -> or6/1
  BrakePedalState/7(output7) -> or7/1
  BrakePedalState/8(output8) -> or8/1
  Steering_Angle_Feedback/1(output1) -> or1/2
  Steering_Angle_Feedback/2(output2) -> or2/2
  Steering_Angle_Feedback/3(output3) -> or3/2
  Steering_Angle_Feedback/4(output4) -> or4/2
  Steering_Angle_Feedback/5(output5) -> or5/2
  Steering_Angle_Feedback/6(output6) -> or6/2
  Steering_Angle_Feedback/7(output7) -> or7/2
  Steering_Angle_Feedback/8(output8) -> or8/2
  Steering_feedback/1(output1) -> or1/3
  Steering_feedback/2(output2) -> or2/3
  Steering_feedback/3(output3) -> or3/3
  Steering_feedback/4(output4) -> or4/3
  Steering_feedback/5(output5) -> or5/3
  Steering_feedback/6(output6) -> or6/3
  Steering_feedback/7(output7) -> or7/3
  Steering_feedback/8(output8) -> or8/3
  Wheel_Speed_RR_Feedback/1(output1) -> or1/4
  Wheel_Speed_RR_Feedback/2(output2) -> or2/4
  Wheel_Speed_RR_Feedback/3(output3) -> or3/4
  Wheel_Speed_RR_Feedback/4(output4) -> or4/4
  Wheel_Speed_RR_Feedback/5(output5) -> or5/4
  Wheel_Speed_RR_Feedback/6(output6) -> or6/4
  Wheel_Speed_RR_Feedback/7(output7) -> or7/4
  Wheel_Speed_RR_Feedback/8(output8) -> or8/4
  Wheel_Speed_RL_Feedback/1(output1) -> or1/5
  Wheel_Speed_RL_Feedback/2(output2) -> or2/5
  Wheel_Speed_RL_Feedback/3(output3) -> or3/5
  Wheel_Speed_RL_Feedback/4(output4) -> or4/5
  Wheel_Speed_RL_Feedback/5(output5) -> or5/5
  Wheel_Speed_RL_Feedback/6(output6) -> or6/5
  Wheel_Speed_RL_Feedback/7(output7) -> or7/5
  Wheel_Speed_RL_Feedback/8(output8) -> or8/5
  Wheel_Speed_FR_Feedback/1(output1) -> or1/6
  Wheel_Speed_FR_Feedback/2(output2) -> or2/6
  Wheel_Speed_FR_Feedback/3(output3) -> or3/6
  Wheel_Speed_FR_Feedback/4(output4) -> or4/6
  Wheel_Speed_FR_Feedback/5(output5) -> or5/6
  Wheel_Speed_FR_Feedback/6(output6) -> or6/6
  Wheel_Speed_FR_Feedback/7(output7) -> or7/6
  Wheel_Speed_FR_Feedback/8(output8) -> or8/6
  Wheel_Speed_FL_Feedback/1(output1) -> or1/7
  Wheel_Speed_FL_Feedback/2(output2) -> or2/7
  Wheel_Speed_FL_Feedback/3(output3) -> or3/7
  Wheel_Speed_FL_Feedback/4(output4) -> or4/7
  Wheel_Speed_FL_Feedback/5(output5) -> or5/7
  Wheel_Speed_FL_Feedback/6(output6) -> or6/7
  Wheel_Speed_FL_Feedback/7(output7) -> or7/7
  Wheel_Speed_FL_Feedback/8(output8) -> or8/7
  or1/1 -> Conv1/1
  Conv1/1 -> VCU2IPC502_mux/1
  or2/1 -> Conv2/1
  Conv2/1 -> VCU2IPC502_mux/2
  or3/1 -> Conv3/1
  Conv3/1 -> VCU2IPC502_mux/3
  or4/1 -> Conv4/1
  Conv4/1 -> VCU2IPC502_mux/4
  or5/1 -> Conv5/1
  Conv5/1 -> VCU2IPC502_mux/5
  or6/1 -> Conv6/1
  Conv6/1 -> VCU2IPC502_mux/6
  or7/1 -> Conv7/1
  Conv7/1 -> VCU2IPC502_mux/7
  or8/1 -> Conv8/1
  Conv8/1 -> VCU2IPC502_mux/8
  VCU2IPC502_ID/1 -> VCU2IPC502_ID_Out/1
  VCU2IPC502_DLC/1 -> VCU2IPC502_DLC_Out/1
  BrakePedalState_in/1 -> BrakePedalState/1(BrakePedalState)
  Steering_Angle_Feedback_in/1 -> Steering_Angle_Feedback/1(Steering_Angle_Feedback)
  Steering_feedback_in/1 -> Steering_feedback/1(Steering_feedback)
  Wheel_Speed_RR_Feedback_in/1 -> Wheel_Speed_RR_Feedback/1(Wheel_Speed_RR_Feedback)
  Wheel_Speed_RL_Feedback_in/1 -> Wheel_Speed_RL_Feedback/1(Wheel_Speed_RL_Feedback)
  Wheel_Speed_FR_Feedback_in/1 -> Wheel_Speed_FR_Feedback/1(Wheel_Speed_FR_Feedback)
  Wheel_Speed_FL_Feedback_in/1 -> Wheel_Speed_FL_Feedback/1(Wheel_Speed_FL_Feedback)

== system VCU_CS75_12_30_test/长安CS75底盘程序，20ms一次/Output/CAN0_Tx/to503/VCU2IPC503 ==
  LongitudinalAcceleration_in : Inport
  YawRate_in : Inport  Port=2
  Conv{1..8} (8 alike) : DataTypeConversion
  LongitudinalAcceleration : Subsystem
  VCU2IPC503_DLC : Constant  Value=8  OutDataTypeStr=uint8
  VCU2IPC503_DLC_Out : Terminator
  VCU2IPC503_ID : Constant  Value=1283  OutDataTypeStr=single
  VCU2IPC503_ID_Out : Terminator
  VCU2IPC503_mux : Mux  Inputs=8
  YawRate : Subsystem
  or{1..8} (8 alike) : simulink/Logic and Bit Operations/Bitwise Operator  logicop=OR  UseBitMask=off  NumInputPorts=2  BitMask=bin2dec('11011001')  BitMaskRealWorld=Stored Integer
  output : Outport
  wires:
  VCU2IPC503_mux/1 -> output/1
  LongitudinalAcceleration/1(output1) -> or1/1
  LongitudinalAcceleration/2(output2) -> or2/1
  LongitudinalAcceleration/3(output3) -> or3/1
  LongitudinalAcceleration/4(output4) -> or4/1
  LongitudinalAcceleration/5(output5) -> or5/1
  LongitudinalAcceleration/6(output6) -> or6/1
  LongitudinalAcceleration/7(output7) -> or7/1
  LongitudinalAcceleration/8(output8) -> or8/1
  YawRate/1(output1) -> or1/2
  YawRate/2(output2) -> or2/2
  YawRate/3(output3) -> or3/2
  YawRate/4(output4) -> or4/2
  YawRate/5(output5) -> or5/2
  YawRate/6(output6) -> or6/2
  YawRate/7(output7) -> or7/2
  YawRate/8(output8) -> or8/2
  or1/1 -> Conv1/1
  Conv1/1 -> VCU2IPC503_mux/1
  or2/1 -> Conv2/1
  Conv2/1 -> VCU2IPC503_mux/2
  or3/1 -> Conv3/1
  Conv3/1 -> VCU2IPC503_mux/3
  or4/1 -> Conv4/1
  Conv4/1 -> VCU2IPC503_mux/4
  or5/1 -> Conv5/1
  Conv5/1 -> VCU2IPC503_mux/5
  or6/1 -> Conv6/1
  Conv6/1 -> VCU2IPC503_mux/6
  or7/1 -> Conv7/1
  Conv7/1 -> VCU2IPC503_mux/7
  or8/1 -> Conv8/1
  Conv8/1 -> VCU2IPC503_mux/8
  VCU2IPC503_ID/1 -> VCU2IPC503_ID_Out/1
  VCU2IPC503_DLC/1 -> VCU2IPC503_DLC_Out/1
  LongitudinalAcceleration_in/1 -> LongitudinalAcceleration/1(LongitudinalAcceleration)
  YawRate_in/1 -> YawRate/1(YawRate)

== system VCU_CS75_12_30_test/长安CS75底盘程序，20ms一次/Output/CAN0_Tx/to511/VCU2IPC ==
  Steering_feedback_in : Inport
  Engine_Feedback_in : Inport  Port=2
  Engine_Feedback2_in : Inport  Port=3
  Res_go_in : Inport  Port=4
  Wheel_Speed_RL_Feedback_in : Inport  Port=5
  Wheel_Speed_RR_Feedback_in : Inport  Port=6
  Steering_Angle_Feedback_in : Inport  Port=7
  Conv{1..8} (8 alike) : DataTypeConversion
  Engine_Feedback : Subsystem
  Engine_Feedback2 : Subsystem
  Res_go : Subsystem
  Steering_Angle_Feedback : Subsystem
  Steering_feedback : Subsystem
  VCU2IPC_DLC : Constant  Value=8  OutDataTypeStr=uint8
  VCU2IPC_DLC_Out : Terminator
  VCU2IPC_ID : Constant  Value=1297  OutDataTypeStr=single
  VCU2IPC_ID_Out : Terminator
  VCU2IPC_mux : Mux  Inputs=8
  Wheel_Speed_RL_Feedback : Subsystem
  Wheel_Speed_RR_Feedback : Subsystem
  or{1..8} (8 alike) : simulink/Logic and Bit Operations/Bitwise Operator  logicop=OR  UseBitMask=off  NumInputPorts=7  BitMask=bin2dec('11011001')  BitMaskRealWorld=Stored Integer
  output : Outport
  wires:
  VCU2IPC_mux/1 -> output/1
  Steering_feedback/1(output1) -> or1/1
  Steering_feedback/2(output2) -> or2/1
  Steering_feedback/3(output3) -> or3/1
  Steering_feedback/4(output4) -> or4/1
  Steering_feedback/5(output5) -> or5/1
  Steering_feedback/6(output6) -> or6/1
  Steering_feedback/7(output7) -> or7/1
  Steering_feedback/8(output8) -> or8/1
  Engine_Feedback/1(output1) -> or1/2
  Engine_Feedback/2(output2) -> or2/2
  Engine_Feedback/3(output3) -> or3/2
  Engine_Feedback/4(output4) -> or4/2
  Engine_Feedback/5(output5) -> or5/2
  Engine_Feedback/6(output6) -> or6/2
  Engine_Feedback/7(output7) -> or7/2
  Engine_Feedback/8(output8) -> or8/2
  Engine_Feedback2/1(output1) -> or1/3
  Engine_Feedback2/2(output2) -> or2/3
  Engine_Feedback2/3(output3) -> or3/3
  Engine_Feedback2/4(output4) -> or4/3
  Engine_Feedback2/5(output5) -> or5/3
  Engine_Feedback2/6(output6) -> or6/3
  Engine_Feedback2/7(output7) -> or7/3
  Engine_Feedback2/8(output8) -> or8/3
  Res_go/1(output1) -> or1/4
  Res_go/2(output2) -> or2/4
  Res_go/3(output3) -> or3/4
  Res_go/4(output4) -> or4/4
  Res_go/5(output5) -> or5/4
  Res_go/6(output6) -> or6/4
  Res_go/7(output7) -> or7/4
  Res_go/8(output8) -> or8/4
  Wheel_Speed_RL_Feedback/1(output1) -> or1/5
  Wheel_Speed_RL_Feedback/2(output2) -> or2/5
  Wheel_Speed_RL_Feedback/3(output3) -> or3/5
  Wheel_Speed_RL_Feedback/4(output4) -> or4/5
  Wheel_Speed_RL_Feedback/5(output5) -> or5/5
  Wheel_Speed_RL_Feedback/6(output6) -> or6/5
  Wheel_Speed_RL_Feedback/7(output7) -> or7/5
  Wheel_Speed_RL_Feedback/8(output8) -> or8/5
  Wheel_Speed_RR_Feedback/1(output1) -> or1/6
  Wheel_Speed_RR_Feedback/2(output2) -> or2/6
  Wheel_Speed_RR_Feedback/3(output3) -> or3/6
  Wheel_Speed_RR_Feedback/4(output4) -> or4/6
  Wheel_Speed_RR_Feedback/5(output5) -> or5/6
  Wheel_Speed_RR_Feedback/6(output6) -> or6/6
  Wheel_Speed_RR_Feedback/7(output7) -> or7/6
  Wheel_Speed_RR_Feedback/8(output8) -> or8/6
  Steering_Angle_Feedback/1(output1) -> or1/7
  Steering_Angle_Feedback/2(output2) -> or2/7
  Steering_Angle_Feedback/3(output3) -> or3/7
  Steering_Angle_Feedback/4(output4) -> or4/7
  Steering_Angle_Feedback/5(output5) -> or5/7
  Steering_Angle_Feedback/6(output6) -> or6/7
  Steering_Angle_Feedback/7(output7) -> or7/7
  Steering_Angle_Feedback/8(output8) -> or8/7
  or1/1 -> Conv1/1
  Conv1/1 -> VCU2IPC_mux/1
  or2/1 -> Conv2/1
  Conv2/1 -> VCU2IPC_mux/2
  or3/1 -> Conv3/1
  Conv3/1 -> VCU2IPC_mux/3
  or4/1 -> Conv4/1
  Conv4/1 -> VCU2IPC_mux/4
  or5/1 -> Conv5/1
  Conv5/1 -> VCU2IPC_mux/5
  or6/1 -> Conv6/1
  Conv6/1 -> VCU2IPC_mux/6
  or7/1 -> Conv7/1
  Conv7/1 -> VCU2IPC_mux/7
  or8/1 -> Conv8/1
  Conv8/1 -> VCU2IPC_mux/8
  VCU2IPC_ID/1 -> VCU2IPC_ID_Out/1
  VCU2IPC_DLC/1 -> VCU2IPC_DLC_Out/1
  Steering_feedback_in/1 -> Steering_feedback/1(Steering_feedback)
  Engine_Feedback_in/1 -> Engine_Feedback/1(Engine_Feedback)
  Engine_Feedback2_in/1 -> Engine_Feedback2/1(Engine_Feedback2)
  Res_go_in/1 -> Res_go/1(Res_go)
  Wheel_Speed_RL_Feedback_in/1 -> Wheel_Speed_RL_Feedback/1(Wheel_Speed_RL_Feedback)
  Wheel_Speed_RR_Feedback_in/1 -> Wheel_Speed_RR_Feedback/1(Wheel_Speed_RR_Feedback)
  Steering_Angle_Feedback_in/1 -> Steering_Angle_Feedback/1(Steering_Angle_Feedback)

== system VCU_CS75_12_30_test/长安CS75底盘程序，20ms一次/Output/CAN0_Tx/to6001/A ==
  Wheel_Speed_RR_Data_in : Inport
  Wheel_Speed_RL_Data_in : Inport  Port=2
  Wheel_Speed_FR_Data_in : Inport  Port=3
  Wheel_Speed_FL_Data_in : Inport  Port=4
  A_DLC : Constant  Value=8  OutDataTypeStr=uint8
  A_DLC_Out : Terminator
  A_ID : Constant  Value=2147508225  OutDataTypeStr=single
  A_ID_Out : Terminator
  A_mux : Mux  Inputs=8
  Conv{1..8} (8 alike) : DataTypeConversion
  Wheel_Speed_FL_Data : Subsystem
  Wheel_Speed_FR_Data : Subsystem
  Wheel_Speed_RL_Data : Subsystem
  Wheel_Speed_RR_Data : Subsystem
  or{1..8} (8 alike) : simulink/Logic and Bit Operations/Bitwise Operator  logicop=OR  UseBitMask=off  NumInputPorts=4  BitMask=bin2dec('11011001')  BitMaskRealWorld=Stored Integer
  output : Outport
  wires:
  Wheel_Speed_FL_Data_in/1 -> Wheel_Speed_FL_Data/1(Wheel_Speed_FL_Data)
  Wheel_Speed_FR_Data_in/1 -> Wheel_Speed_FR_Data/1(Wheel_Speed_FR_Data)
  Wheel_Speed_RL_Data_in/1 -> Wheel_Speed_RL_Data/1(Wheel_Speed_RL_Data)
  Wheel_Speed_RR_Data_in/1 -> Wheel_Speed_RR_Data/1(Wheel_Speed_RR_Data)
  A_DLC/1 -> A_DLC_Out/1
  A_ID/1 -> A_ID_Out/1
  Conv8/1 -> A_mux/8
  or8/1 -> Conv8/1
  Conv7/1 -> A_mux/7
  or7/1 -> Conv7/1
  Conv6/1 -> A_mux/6
  or6/1 -> Conv6/1
  Conv5/1 -> A_mux/5
  or5/1 -> Conv5/1
  Conv4/1 -> A_mux/4
  or4/1 -> Conv4/1
  Conv3/1 -> A_mux/3
  or3/1 -> Conv3/1
  Conv2/1 -> A_mux/2
  or2/1 -> Conv2/1
  Conv1/1 -> A_mux/1
  or1/1 -> Conv1/1
  Wheel_Speed_FL_Data/8(output8) -> or8/4
  Wheel_Speed_FL_Data/7(output7) -> or7/4
  Wheel_Speed_FL_Data/6(output6) -> or6/4
  Wheel_Speed_FL_Data/5(output5) -> or5/4
  Wheel_Speed_FL_Data/4(output4) -> or4/4
  Wheel_Speed_FL_Data/3(output3) -> or3/4
  Wheel_Speed_FL_Data/2(output2) -> or2/4
  Wheel_Speed_FL_Data/1(output1) -> or1/4
  Wheel_Speed_FR_Data/8(output8) -> or8/3
  Wheel_Speed_FR_Data/7(output7) -> or7/3
  Wheel_Speed_FR_Data/6(output6) -> or6/3
  Wheel_Speed_FR_Data/5(output5) -> or5/3
  Wheel_Speed_FR_Data/4(output4) -> or4/3
  Wheel_Speed_FR_Data/3(output3) -> or3/3
  Wheel_Speed_FR_Data/2(output2) -> or2/3
  Wheel_Speed_FR_Data/1(output1) -> or1/3
  Wheel_Speed_RL_Data/8(output8) -> or8/2
  Wheel_Speed_RL_Data/7(output7) -> or7/2
  Wheel_Speed_RL_Data/6(output6) -> or6/2
  Wheel_Speed_RL_Data/5(output5) -> or5/2
  Wheel_Speed_RL_Data/4(output4) -> or4/2
  Wheel_Speed_RL_Data/3(output3) -> or3/2
  Wheel_Speed_RL_Data/2(output2) -> or2/2
  Wheel_Speed_RL_Data/1(output1) -> or1/2
  Wheel_Speed_RR_Data/8(output8) -> or8/1
  Wheel_Speed_RR_Data/7(output7) -> or7/1
  Wheel_Speed_RR_Data/6(output6) -> or6/1
  Wheel_Speed_RR_Data/5(output5) -> or5/1
  Wheel_Speed_RR_Data/4(output4) -> or4/1
  Wheel_Speed_RR_Data/3(output3) -> or3/1
  Wheel_Speed_RR_Data/2(output2) -> or2/1
  Wheel_Speed_RR_Data/1(output1) -> or1/1
  A_mux/1 -> output/1

== system VCU_CS75_12_30_test/长安CS75底盘程序，20ms一次/Output/CAN0_Tx/to6002/B ==
  RemoteDecelerationRequest_in : Inport
  RemoteThrottlePercentage_in : Inport  Port=2
  BrakePeadlState_in : Inport  Port=3
  ThrottlePedalPercentage_in : Inport  Port=4
  Steering_Angle_in : Inport  Port=5
  VehicleSpeed_in : Inport  Port=6
  B_DLC : Constant  Value=8  OutDataTypeStr=uint8
  B_DLC_Out : Terminator
  B_ID : Constant  Value=2147508226  OutDataTypeStr=single
  B_ID_Out : Terminator
  B_mux : Mux  Inputs=8
  BrakePeadlState : Subsystem
  Conv{1..8} (8 alike) : DataTypeConversion
  RemoteDecelerationRequest : Subsystem
  RemoteThrottlePercentage : Subsystem
  Steering_Angle : Subsystem
  ThrottlePedalPercentage : Subsystem
  VehicleSpeed : Subsystem
  or{1..8} (8 alike) : simulink/Logic and Bit Operations/Bitwise Operator  logicop=OR  UseBitMask=off  NumInputPorts=6  BitMask=bin2dec('11011001')  BitMaskRealWorld=Stored Integer
  output : Outport
  wires:
  B_mux/1 -> output/1
  RemoteDecelerationRequest/1(output1) -> or1/1
  RemoteDecelerationRequest/2(output2) -> or2/1
  RemoteDecelerationRequest/3(output3) -> or3/1
  RemoteDecelerationRequest/4(output4) -> or4/1
  RemoteDecelerationRequest/5(output5) -> or5/1
  RemoteDecelerationRequest/6(output6) -> or6/1
  RemoteDecelerationRequest/7(output7) -> or7/1
  RemoteDecelerationRequest/8(output8) -> or8/1
  RemoteThrottlePercentage/1(output1) -> or1/2
  RemoteThrottlePercentage/2(output2) -> or2/2
  RemoteThrottlePercentage/3(output3) -> or3/2
  RemoteThrottlePercentage/4(output4) -> or4/2
  RemoteThrottlePercentage/5(output5) -> or5/2
  RemoteThrottlePercentage/6(output6) -> or6/2
  RemoteThrottlePercentage/7(output7) -> or7/2
  RemoteThrottlePercentage/8(output8) -> or8/2
  BrakePeadlState/1(output1) -> or1/3
  BrakePeadlState/2(output2) -> or2/3
  BrakePeadlState/3(output3) -> or3/3
  BrakePeadlState/4(output4) -> or4/3
  BrakePeadlState/5(output5) -> or5/3
  BrakePeadlState/6(output6) -> or6/3
  BrakePeadlState/7(output7) -> or7/3
  BrakePeadlState/8(output8) -> or8/3
  ThrottlePedalPercentage/1(output1) -> or1/4
  ThrottlePedalPercentage/2(output2) -> or2/4
  ThrottlePedalPercentage/3(output3) -> or3/4
  ThrottlePedalPercentage/4(output4) -> or4/4
  ThrottlePedalPercentage/5(output5) -> or5/4
  ThrottlePedalPercentage/6(output6) -> or6/4
  ThrottlePedalPercentage/7(output7) -> or7/4
  ThrottlePedalPercentage/8(output8) -> or8/4
  Steering_Angle/1(output1) -> or1/5
  Steering_Angle/2(output2) -> or2/5
  Steering_Angle/3(output3) -> or3/5
  Steering_Angle/4(output4) -> or4/5
  Steering_Angle/5(output5) -> or5/5
  Steering_Angle/6(output6) -> or6/5
  Steering_Angle/7(output7) -> or7/5
  Steering_Angle/8(output8) -> or8/5
  VehicleSpeed/1(output1) -> or1/6
  VehicleSpeed/2(output2) -> or2/6
  VehicleSpeed/3(output3) -> or3/6
  VehicleSpeed/4(output4) -> or4/6
  VehicleSpeed/5(output5) -> or5/6
  VehicleSpeed/6(output6) -> or6/6
  VehicleSpeed/7(output7) -> or7/6
  VehicleSpeed/8(output8) -> or8/6
  or1/1 -> Conv1/1
  Conv1/1 -> B_mux/1
  or2/1 -> Conv2/1
  Conv2/1 -> B_mux/2
  or3/1 -> Conv3/1
  Conv3/1 -> B_mux/3
  or4/1 -> Conv4/1
  Conv4/1 -> B_mux/4
  or5/1 -> Conv5/1
  Conv5/1 -> B_mux/5
  or6/1 -> Conv6/1
  Conv6/1 -> B_mux/6
  or7/1 -> Conv7/1
  Conv7/1 -> B_mux/7
  or8/1 -> Conv8/1
  Conv8/1 -> B_mux/8
  B_ID/1 -> B_ID_Out/1
  B_DLC/1 -> B_DLC_Out/1
  RemoteDecelerationRequest_in/1 -> RemoteDecelerationRequest/1(RemoteDecelerationRequest)
  RemoteThrottlePercentage_in/1 -> RemoteThrottlePercentage/1(RemoteThrottlePercentage)
  BrakePeadlState_in/1 -> BrakePeadlState/1(BrakePeadlState)
  ThrottlePedalPercentage_in/1 -> ThrottlePedalPercentage/1(ThrottlePedalPercentage)
  Steering_Angle_in/1 -> Steering_Angle/1(Steering_Angle)
  VehicleSpeed_in/1 -> VehicleSpeed/1(VehicleSpeed)
